simulink model "first_order"  (R2020b)
settings: Solver=VariableStepAuto  StartTime=0.0  StopTime=10.0  RelTol=1e-3
libraries: simulink x1
settings Model: Creator=adima  LastModifiedBy=adima

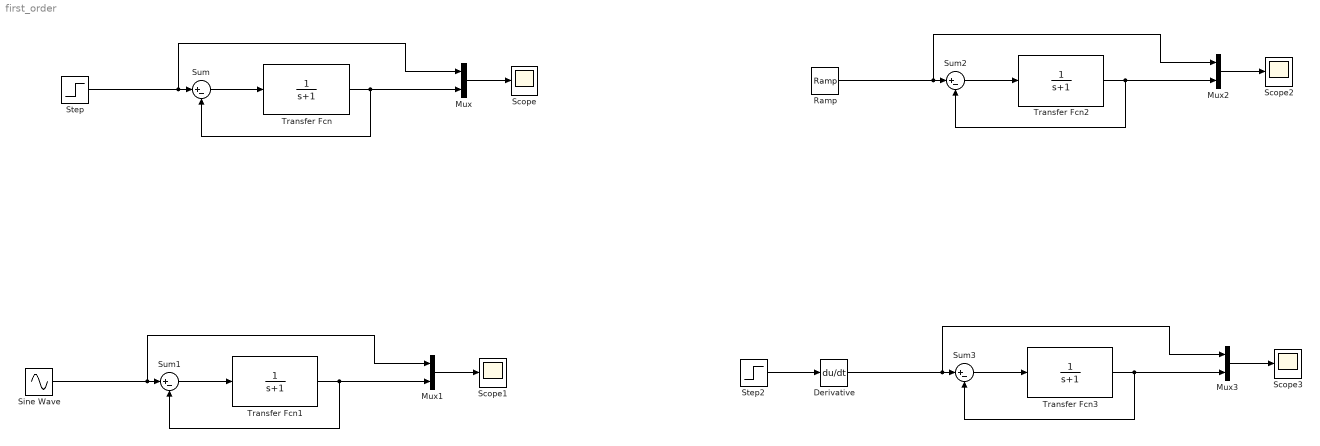
== system first_order ==
  Derivative : Derivative
  Mux{,1..3} (4 alike) : Mux  Inputs=2
  Ramp : simulink/Sources/Ramp  slope=1  start=0  InitialOutput=0
  Scope{,1..3} (4 alike) : Scope
  Sine Wave : Sin  SampleTime=0
  Step : Step  SampleTime=0
  Step2 : Step  SampleTime=0
  Sum{,1..3} (4 alike) : Sum  Inputs=|+-
  Transfer Fcn{,1..3} (4 alike) : TransferFcn  Denominator=[1 1 ]
  wires:
  Step/1 -> Mux/1, Sum/1
  Mux/1 -> Scope/1
  Transfer Fcn/1 -> Mux/2, Sum/2
  Sum/1 -> Transfer Fcn/1
  Transfer Fcn1/1 -> Mux1/2, Sum1/2
  Sum1/1 -> Transfer Fcn1/1
  Mux1/1 -> Scope1/1
  Sine Wave/1 -> Mux1/1, Sum1/1
  Transfer Fcn2/1 -> Mux2/2, Sum2/2
  Sum2/1 -> Transfer Fcn2/1
  Mux2/1 -> Scope2/1
  Ramp/1 -> Mux2/1, Sum2/1
  Transfer Fcn3/1 -> Mux3/2, Sum3/2
  Sum3/1 -> Transfer Fcn3/1
  Mux3/1 -> Scope3/1
  Derivative/1 -> Mux3/1, Sum3/1
  Step2/1 -> Derivative/1
